simulink model "acquisition"  (R2020a)
settings: Solver=VariableStepAuto  StartTime=0.0  StopTime=simulation_time  RelTol=1e-3
values from neighbouring files (symbols this model uses):
  ca_fft_coef = zeros(37,4096)    [acquisition_hw_init.m]
  ca_fft_width = 14    [acquisition_hw_init.m]
  core_upsample_ratio = 24    [acquisition_hw_init.m]
  correlator_latency = 19    [acquisition_hw_init.m]
  ddc_latency = 5    [acquisition_hw_init.m]
  DDS_signal_width = 12    [acquisition_hw_init.m]
  f_start_phase = core_upsample_ratio*f_start/fs    (= -0.0006103515625)    [acquisition_hw_init.m]
  fd_phase_increment = core_upsample_ratio*(f_dds_change)/fs    (= 2e-05)    [acquisition_hw_init.m]
  fft_length = 4096    [acquisition_hw_init.m]
  fs = core_upsample_ratio*fs_adc    (= 120000000)    [acquisition_hw_init.m]
  ts = 1/fs    [acquisition_debugger_data.m]    (also in acquisition_hw_init.m = 8.33333333333e-09)
  ts_adc = 1/fs_adc    (= 2e-07)    [acquisition_hw_init.m]
libraries: xbsIndex_r4 x325
(part 2 of 2)

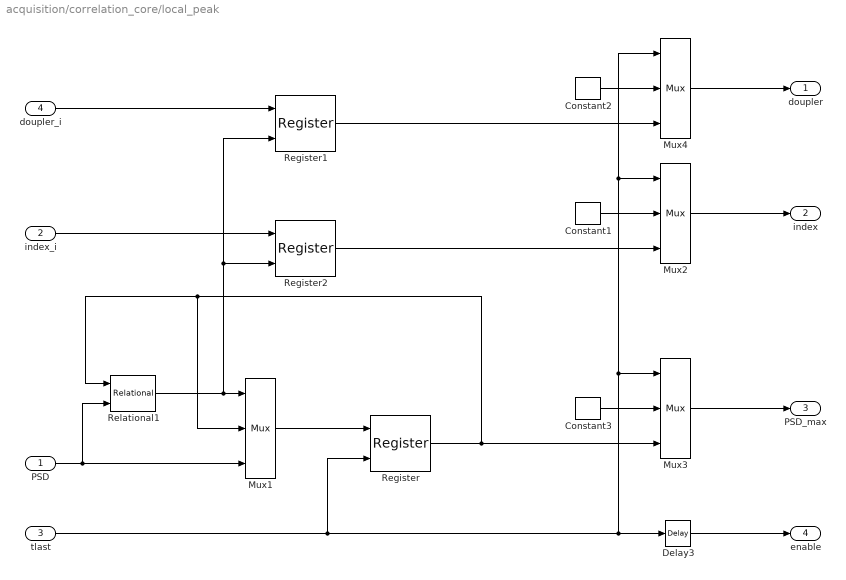
== system acquisition/correlation_core/local_peak ==
  PSD : Inport
  index_i : Inport  Port=2
  tlast : Inport  Port=3
  doupler_i : Inport  Port=4
  Constant1 : xbsIndex_r4/Constant  const=0  gui_display_data_type=Fixed-point  arith_type=Unsigned  n_bits=1  bin_pt=0  preci_type=Single  exp_width=8  frac_width=24  explicit_period=on  period=ts  equ=P=C  opselect=C  inp2=PCIN>>17  opr=+  inp1=P  carry=CIN  dbl_ovrd=off  block_type=constant
  Constant2 : xbsIndex_r4/Constant  const=0  gui_display_data_type=Fixed-point  arith_type=Unsigned  n_bits=DDS_phase_width  bin_pt=DDS_phase_width  preci_type=Single  exp_width=8  frac_width=24  explicit_period=on  period=ts  equ=P=C  opselect=C  inp2=PCIN>>17  opr=+  inp1=P  carry=CIN  dbl_ovrd=off  block_type=constant
  Constant3 : xbsIndex_r4/Constant  const=0  gui_display_data_type=Fixed-point  arith_type=Unsigned  n_bits=1  bin_pt=0  preci_type=Single  exp_width=8  frac_width=24  explicit_period=on  period=ts  equ=P=C  opselect=C  inp2=PCIN>>17  opr=+  inp1=P  carry=CIN  dbl_ovrd=off  block_type=constant
  Delay3 : xbsIndex_r4/Delay  rst=off  infoeditControl=Selection of Reset will increase slice count due to use of real FFs and instead of SRLs  en=off  latency=1  reg_retiming=off  dbl_ovrd=off  block_type=delay
  Mux1 : xbsIndex_r4/Mux  inputs=2  en=off  latency=0  precision=Full  arith_type=Unsigned  n_bits=16  bin_pt=14  quantization=Truncate  overflow=Wrap  dbl_ovrd=off  block_type=mux
  Mux2 : xbsIndex_r4/Mux  inputs=2  en=off  latency=1  precision=Full  arith_type=Unsigned  n_bits=16  bin_pt=14  quantization=Truncate  overflow=Wrap  dbl_ovrd=off  block_type=mux
  Mux3 : xbsIndex_r4/Mux  inputs=2  en=off  latency=1  precision=Full  arith_type=Unsigned  n_bits=16  bin_pt=14  quantization=Truncate  overflow=Wrap  dbl_ovrd=off  block_type=mux
  Mux4 : xbsIndex_r4/Mux  inputs=2  en=off  latency=1  precision=Full  arith_type=Unsigned  n_bits=16  bin_pt=14  quantization=Truncate  overflow=Wrap  dbl_ovrd=off  block_type=mux
  Register : xbsIndex_r4/Register  init=-2048  rst=on  en=off  dbl_ovrd=off  block_type=register
  Register1 : xbsIndex_r4/Register  init=0  rst=off  en=on  dbl_ovrd=off  block_type=register
  Register2 : xbsIndex_r4/Register  init=0  rst=off  en=on  dbl_ovrd=off  block_type=register
  Relational1 : xbsIndex_r4/Relational  mode=a<b  op_type=Bool  en=off  latency=0  dbl_ovrd=off  block_type=relational
  doupler : Outport
  index : Outport  Port=2
  PSD_max : Outport  Port=3
  enable : Outport  Port=4
  wires:
  Constant3/1 -> Mux3/2
  Constant1/1 -> Mux2/2
  Register2/1 -> Mux2/3
  Register/1 -> Relational1/1, Mux1/2, Mux3/3
  index_i/1 -> Register2/1
  Mux1/1 -> Register/1
  Relational1/1 -> Mux1/1, Register1/2, Register2/2
  PSD/1 -> Relational1/2, Mux1/3
  tlast/1 -> Register/2, Mux4/1, Mux2/1, Mux3/1, Delay3/1
  Delay3/1 -> enable/1
  Mux2/1 -> index/1
  Mux3/1 -> PSD_max/1
  doupler_i/1 -> Register1/1
  Constant2/1 -> Mux4/2
  Register1/1 -> Mux4/3
  Mux4/1 -> doupler/1

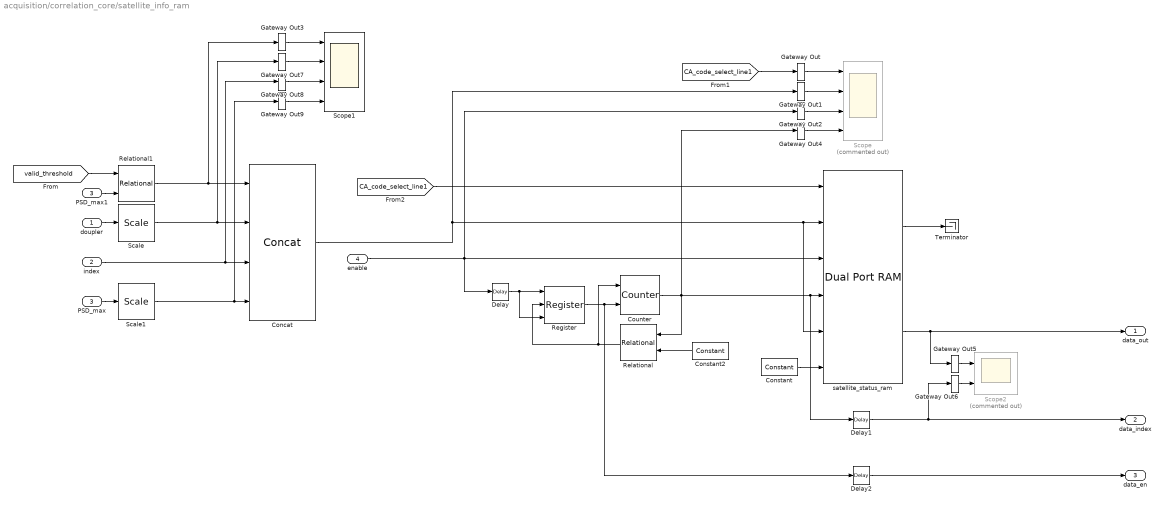
== system acquisition/correlation_core/satellite_info_ram ==
  doupler : Inport
  index : Inport  Port=2
  PSD_max : Inport  Port=3
  enable : Inport  Port=4
  Concat : xbsIndex_r4/Concat  num_inputs=4  dbl_ovrd=off  block_type=concat
  Constant : xbsIndex_r4/Constant  const=0  gui_display_data_type=Boolean  arith_type=Boolean  n_bits=16  bin_pt=14  preci_type=Single  exp_width=8  frac_width=24  explicit_period=on  period=ts  equ=P=C  opselect=C  inp2=PCIN>>17  opr=+  inp1=P  carry=CIN  dbl_ovrd=off  block_type=constant
  Constant2 : xbsIndex_r4/Constant  const=36  gui_display_data_type=Fixed-point  arith_type=Unsigned  n_bits=ceil(log2(37))  bin_pt=0  preci_type=Single  exp_width=8  frac_width=24  explicit_period=on  period=ts  equ=P=C  opselect=C  inp2=PCIN>>17  opr=+  inp1=P  carry=CIN  dbl_ovrd=off  block_type=constant
  Counter : xbsIndex_r4/Counter  cnt_type=Free Running  cnt_to=Inf  operation=Up  start_count=0  cnt_by_val=1  arith_type=Unsigned  n_bits=ceil(log2(37))  bin_pt=0  load_pin=off  rst=on  en=on  explicit_period=off  period=1  use_behavioral_HDL=off  implementation=Fabric  dbl_ovrd=off  block_type=counter
  Delay : xbsIndex_r4/Delay  rst=off  infoeditControl=Selection of Reset will increase slice count due to use of real FFs and instead of SRLs  en=off  latency=14  reg_retiming=off  dbl_ovrd=off  block_type=delay
  Delay1 : xbsIndex_r4/Delay  rst=off  infoeditControl=Selection of Reset will increase slice count due to use of real FFs and instead of SRLs  en=off  latency=1  reg_retiming=off  dbl_ovrd=off  block_type=delay
  Delay2 : xbsIndex_r4/Delay  rst=off  infoeditControl=Selection of Reset will increase slice count due to use of real FFs and instead of SRLs  en=off  latency=2  reg_retiming=off  dbl_ovrd=off  block_type=delay
  Gateway Out{,1..9} (10 alike) : xbsIndex_r4/Gateway Out  inherit_from_input=off  hdl_port=off  rows=1  columns=1  UseAsDAC=off  DACChannel='1'  interface=None  automatic_assignment=on  address_offset=hex2dec('00')  intf_name=''  intf_description=''  timing_constraint=None  locs_specified=off  LOCs={}  io_standard={}  block_type=gatewayout
  PSD_max1 : InportShadow  Port=3
  Register : xbsIndex_r4/Register  init=0  rst=on  en=on  dbl_ovrd=off  block_type=register
  Relational : xbsIndex_r4/Relational  mode=a>=b  op_type=Bool  en=off  latency=0  dbl_ovrd=off  block_type=relational
  Relational1 : xbsIndex_r4/Relational  mode=a<=b  op_type=Bool  en=off  latency=0  dbl_ovrd=off  block_type=relational
  Scale : xbsIndex_r4/Scale  scale_factor=DDS_phase_width  dbl_ovrd=off  block_type=scale
  Scale1 : xbsIndex_r4/Scale  scale_factor=abs_adder_point  dbl_ovrd=off  block_type=scale
  Scope : Scope  Commented=on  NumInputPorts=4
  Scope1 : Scope  NumInputPorts=4
  Scope2 : Scope  Commented=on  NumInputPorts=2
  Terminator : Terminator
  satellite_status_ram : xbsIndex_r4/Dual Port RAM  depth=37  initVector=1:37  distributed_mem=Block RAM  init_a=0  init_b=0  rst_a=off  rst_b=off  en_a=off  en_b=off  latency=1  write_mode_A=Read After Write  write_mode_B=Read After Write  optimize=Area  dbl_ovrd=off  simulation_type=fast_sim  block_type=dpram
  data_out : Outport
  data_index : Outport  Port=2
  data_en : Outport  Port=3
  wires:
  [CA_code_select_line1] -> satellite_status_ram/1
  PSD_max/1 -> Scale1/1
  enable/1 -> satellite_status_ram/3, Delay/1, Gateway Out2/1
  Scale/1 -> Gateway Out7/1, Concat/2
  doupler/1 -> Scale/1
  Gateway Out4/1 -> Scope/4
  Gateway Out1/1 -> Scope/2
  Gateway Out/1 -> Scope/1
  Gateway Out2/1 -> Scope/3
  [CA_code_select_line1] -> Gateway Out/1
  Constant/1 -> satellite_status_ram/6
  Concat/1 -> Gateway Out1/1, satellite_status_ram/5, satellite_status_ram/2
  Counter/1 -> Gateway Out4/1, Relational/1, Delay1/1, satellite_status_ram/4
  Register/1 -> Delay2/1, Counter/2
  Delay/1 -> Register/1, Register/3
  Relational/1 -> Counter/1, Register/2
  Constant2/1 -> Relational/2
  Gateway Out5/1 -> Scope2/1
  Gateway Out6/1 -> Scope2/2
  satellite_status_ram/2 -> data_out/1, Gateway Out5/1
  Delay1/1 -> data_index/1, Gateway Out6/1
  satellite_status_ram/1 -> Terminator/1
  Delay2/1 -> data_en/1
  index/1 -> Gateway Out8/1, Concat/3
  Scale1/1 -> Gateway Out9/1, Concat/4
  Relational1/1 -> Gateway Out3/1, Concat/1
  [valid_threshold] -> Relational1/1
  PSD_max1/1 -> Relational1/2
  Gateway Out8/1 -> Scope1/3
  Gateway Out3/1 -> Scope1/1
  Gateway Out7/1 -> Scope1/2
  Gateway Out9/1 -> Scope1/4

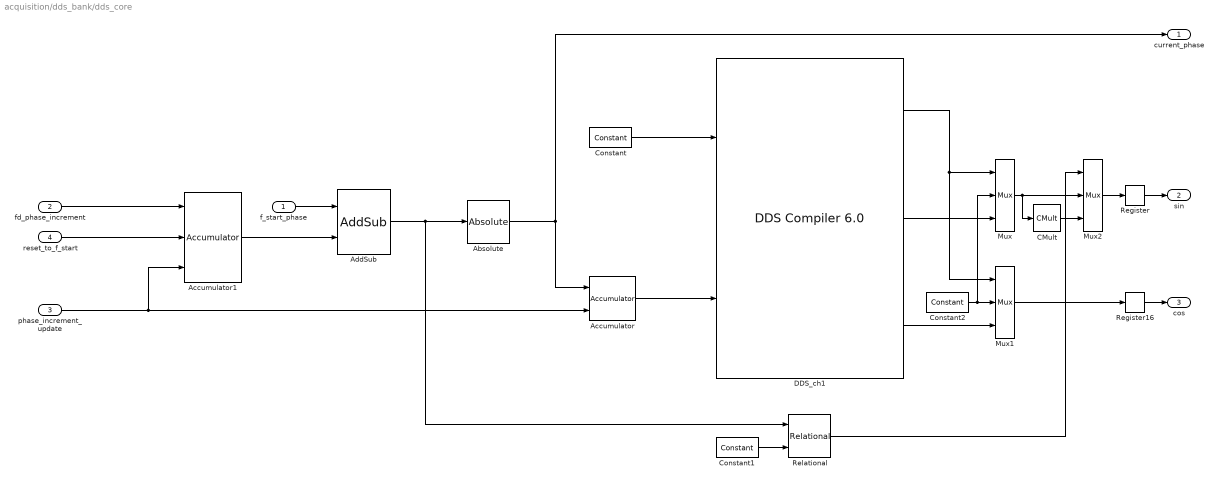
== system acquisition/dds_bank/dds_core ==
  f_start_phase : Inport
  fd_phase_increment : Inport  Port=2
  phase_increment_update : Inport  Port=3
  reset_to_f_start : Inport  Port=4
  Absolute : xbsIndex_r4/Absolute  precision=User Defined  arith_type=Unsigned  n_bits=DDS_phase_width  bin_pt=DDS_phase_width  quantization="Round  (unbiased: +/- Inf)"  overflow=Saturate  en=off  latency=0  dbl_ovrd=off  block_type=abs
  Accumulator : xbsIndex_r4/Accumulator  operation=Add  n_bits=DDS_phase_width  overflow=Wrap  scale=1  rst=on  hasbypass=off  infoeditControl=reset for floating point data type must be asserted for a minimum of 2 cycles  en=off  latency=1  msb_inp=100  msb=100  lsb=-100  use_behavioral_HDL=on  implementation=Fabric  dbl_ovrd=off  block_type=accum
  Accumulator1 : xbsIndex_r4/Accumulator  operation=Add  n_bits=DDS_phase_width  overflow=Wrap  scale=1  rst=on  hasbypass=off  infoeditControl=reset for floating point data type must be asserted for a minimum of 2 cycles  en=on  latency=1  msb_inp=100  msb=100  lsb=-100  use_behavioral_HDL=on  implementation=Fabric  dbl_ovrd=off  block_type=accum
  AddSub : xbsIndex_r4/AddSub  mode=Addition  use_carryin=off  use_carryout=off  en=off  latency=1  precision=Full  arith_type=Unsigned  n_bits=DDS_phase_width  bin_pt=DDS_phase_width  quantization="Round  (unbiased: +/- Inf)"  overflow=Saturate  use_behavioral_HDL=off  hw_selection=Fabric  pipelined=off  dbl_ovrd=off  block_type=addsub
  CMult : xbsIndex_r4/CMult  const=-1  gui_display_data_type=Fixed-point  const_n_bits=1  const_bin_pt=0  float_type=Single  exp_bits=8  fraction_bits=24  en=off  latency=0  precision=User Defined  arith_type="Signed  (2's comp)"  n_bits=DDS_signal_width  bin_pt=DDS_signal_width-1  quantization="Round  (unbiased: +/- Inf)"  overflow=Saturate  use_behavioral_HDL=off  mem_type=Distributed RAM  pipeline=off  dbl_ovrd=off  block_type=cmult
  Constant : xbsIndex_r4/Constant  const=1.0  gui_display_data_type=Boolean  arith_type=Boolean  n_bits=16  bin_pt=14  preci_type=Single  exp_width=8  frac_width=24  explicit_period=on  period=ts  equ=P=C  opselect=C  inp2=PCIN>>17  opr=+  inp1=P  carry=CIN  dbl_ovrd=off  block_type=constant
  Constant1 : xbsIndex_r4/Constant  const=0  gui_display_data_type=Fixed-point  arith_type=Unsigned  n_bits=1  bin_pt=0  preci_type=Single  exp_width=8  frac_width=24  explicit_period=on  period=ts  equ=P=C  opselect=C  inp2=PCIN>>17  opr=+  inp1=P  carry=CIN  dbl_ovrd=off  block_type=constant
  Constant2 : xbsIndex_r4/Constant  const=0  gui_display_data_type=Fixed-point  arith_type=Unsigned  n_bits=1  bin_pt=0  preci_type=Single  exp_width=8  frac_width=24  explicit_period=on  period=ts  equ=P=C  opselect=C  inp2=PCIN>>17  opr=+  inp1=P  carry=CIN  dbl_ovrd=off  block_type=constant
  DDS_ch1 : xbsIndex_r4/DDS Compiler 6.0   partspresent=SIN_COS_LUT_only  dds_clock_rate=100  channels=1  mode_of_operation=Standard  modulus=9  parameter_entry=Hardware_Parameters  spurious_free_dynamic_range=45  frequency_resolution=0.4  noise_shaping=Taylor_Series_Corrected  phase_width=DDS_phase_width  output_width=DDS_signal_width  output_selection=Sine_and_Cosine  negative_sine=off  negative_cosine=off  amplitude_mode=Full_Range  memory_type=Auto  optimization_goal=Auto  dsp48_use=Minimal  resync=off  latency_configuration=Auto  latency=1  has_phase_out=off  has_aclken=off  has_aresetn=off  explicit_period=off  period=1  data_has_tlast=Not_Required  has_tready=off  s_phase_has_tuser=Not_Required  m_data_has_tuser=Not_Required  m_phase_has_tuser=Not_Required  s_phase_tuser_width=1  output_form=Twos_Complement  s_config_sync_mode=On_Vector  phase_increment=Programmable  output_frequency1=0  output_frequency2=0  output_frequency3=0  output_frequency4=0  output_frequency5=0  output_frequency6=0  output_frequency7=0  output_frequency8=0  output_frequency9=0  output_frequency10=0  output_frequency11=0  output_frequency12=0  output_frequency13=0  output_frequency14=0  output_frequency15=0  output_frequency16=0  pinc1='0'  pinc2='0'  pinc3='0'  pinc4='0'  pinc5='0'  pinc6='0'  pinc7='0'  pinc8='0'  pinc9='0'  pinc10='0'  pinc11='0'  pinc12='0'  pinc13='0'  pinc14='0'  pinc15='0'  pinc16='0'  phase_offset=None  phase_offset_angles1=0  phase_offset_angles2=0  phase_offset_angles3=0  phase_offset_angles4=0  phase_offset_angles5=0  phase_offset_angles6=0  phase_offset_angles7=0  phase_offset_angles8=0  phase_offset_angles9=0  phase_offset_angles10=0  phase_offset_angles11=0  phase_offset_angles12=0  phase_offset_angles13=0  phase_offset_angles14=0  phase_offset_angles15=0  phase_offset_angles16=0  poff1='0'  poff2='0'  poff3='0'  poff4='0'  poff5='0'  poff6='0'  poff7='0'  poff8='0'  poff9='0'  poff10='0'  poff11='0'  poff12='0'  poff13='0'  poff14='0'  poff15='0'  poff16='0'  trim_axipin_name=on  simulation_type=hybrid_sim  simulation_model=sysgen:xddsv6_0_cmodel  data_path_portlist={ 's_axis_config_tdata_poff', 's_axis_config_tdata_chan0_poff', 's_axis_config_tdata_pinc', 's_axis_config_tdata_chan0_pinc', 's_axis_phase_tdata_resync', 's_axis_phase_tdata_chan0_resync', 's_axis_phase_tdata_poff', 's_axis_phase_tdata_chan0_poff', 's_axis_phase_tdata_pinc', 's_axis_phase_tdata_chan0_pinc', 's_axis_phase_tdata_phase_in', 'm_axis_data_tdata_sine', 'm_axis_data_tdata_chan0_sine', 'm_axis_data_tdata_cosine', 'm_axis_data_tdata_chan0_cosine', 'm_axis_phase_tdata_phase_out', 'm_axis_phase_tdata_chan0_phase_out'}  por_mode=false  gui_behaviour=Sysgen  ip_name=DDS Compiler  ip_version=6.0  dsptool_ready=true  wrapper_available=true  port_translation_map={ 'aclken' => 'en', 'aresetn' => 'rst' }  ipcore_usecache=true  ipcore_useipmodelcache=true  ipcore_xco_need_fpga_part=true  ipcore_verbose=false  block_type=dds_compiler_v6_0
  Mux : xbsIndex_r4/Mux  inputs=2  en=off  latency=1  precision=Full  arith_type=Unsigned  n_bits=16  bin_pt=14  quantization=Truncate  overflow=Wrap  dbl_ovrd=off  block_type=mux
  Mux1 : xbsIndex_r4/Mux  inputs=2  en=off  latency=1  precision=Full  arith_type=Unsigned  n_bits=16  bin_pt=14  quantization=Truncate  overflow=Wrap  dbl_ovrd=off  block_type=mux
  Mux2 : xbsIndex_r4/Mux  inputs=2  en=off  latency=0  precision=Full  arith_type=Unsigned  n_bits=16  bin_pt=14  quantization=Truncate  overflow=Wrap  dbl_ovrd=off  block_type=mux
  Register : xbsIndex_r4/Register  init=0  rst=off  en=off  dbl_ovrd=off  block_type=register
  Register16 : xbsIndex_r4/Register  init=0  rst=off  en=off  dbl_ovrd=off  block_type=register
  Relational : xbsIndex_r4/Relational  mode=a<b  op_type=Bool  en=off  latency=1  dbl_ovrd=off  block_type=relational
  current_phase : Outport
  sin : Outport  Port=2
  cos : Outport  Port=3
  wires:
  Mux/1 -> CMult/1, Mux2/2
  Mux1/1 -> Register16/1
  Constant/1 -> DDS_ch1/1
  reset_to_f_start/1 -> Accumulator1/2
  DDS_ch1/2 -> Mux/3
  DDS_ch1/3 -> Mux1/3
  Constant2/1 -> Mux/2, Mux1/2
  DDS_ch1/1 -> Mux1/1, Mux/1
  Accumulator/1 -> DDS_ch1/2
  phase_increment_update/1 -> Accumulator1/3, Accumulator/2
  AddSub/1 -> Relational/1, Absolute/1
  f_start_phase/1 -> AddSub/1
  fd_phase_increment/1 -> Accumulator1/1
  Accumulator1/1 -> AddSub/2
  Mux2/1 -> Register/1
  CMult/1 -> Mux2/3
  Constant1/1 -> Relational/2
  Absolute/1 -> Accumulator/1, current_phase/1
  Relational/1 -> Mux2/1
  Register/1 -> sin/1
  Register16/1 -> cos/1

== system acquisition/adc_dual_buffer/adc_addr_gen1/RE ==
  In : Inport
  Inverter : xbsIndex_r4/Inverter  en=off  latency=1  dbl_ovrd=off  block_type=inv
  Logical1 : xbsIndex_r4/Logical  logical_function=AND  inputs=2  en=off  latency=0  precision=Full  arith_type=Unsigned  n_bits=16  bin_pt=0  align_bp=on  dbl_ovrd=off  block_type=logical
  Out : Outport
  wires:
  Inverter/1 -> Logical1/2
  In/1 -> Inverter/1, Logical1/1
  Logical1/1 -> Out/1

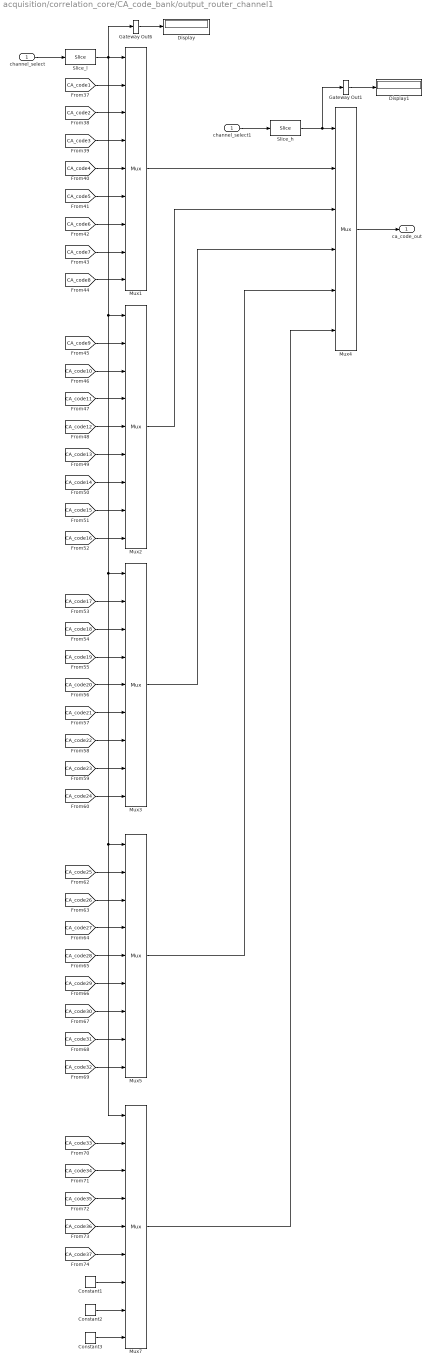
== system acquisition/correlation_core/CA_code_bank/output_router_channel1 ==
  channel_select : Inport
  Constant1 : xbsIndex_r4/Constant  const=0  gui_display_data_type=Fixed-point  arith_type=Unsigned  n_bits=1  bin_pt=0  preci_type=Single  exp_width=8  frac_width=24  explicit_period=on  period=ts  equ=P=C  opselect=C  inp2=PCIN>>17  opr=+  inp1=P  carry=CIN  dbl_ovrd=off  block_type=constant
  Constant2 : xbsIndex_r4/Constant  const=0  gui_display_data_type=Fixed-point  arith_type=Unsigned  n_bits=1  bin_pt=0  preci_type=Single  exp_width=8  frac_width=24  explicit_period=on  period=ts  equ=P=C  opselect=C  inp2=PCIN>>17  opr=+  inp1=P  carry=CIN  dbl_ovrd=off  block_type=constant
  Constant3 : xbsIndex_r4/Constant  const=0  gui_display_data_type=Fixed-point  arith_type=Unsigned  n_bits=1  bin_pt=0  preci_type=Single  exp_width=8  frac_width=24  explicit_period=on  period=ts  equ=P=C  opselect=C  inp2=PCIN>>17  opr=+  inp1=P  carry=CIN  dbl_ovrd=off  block_type=constant
  Display : Display
  Display1 : Display
  Gateway Out1 : xbsIndex_r4/Gateway Out  inherit_from_input=off  hdl_port=off  rows=1  columns=1  UseAsDAC=off  DACChannel='1'  interface=None  automatic_assignment=on  address_offset=hex2dec('00')  intf_name=''  intf_description=''  timing_constraint=None  locs_specified=off  LOCs={}  io_standard={}  block_type=gatewayout
  Gateway Out6 : xbsIndex_r4/Gateway Out  inherit_from_input=off  hdl_port=off  rows=1  columns=1  UseAsDAC=off  DACChannel='1'  interface=None  automatic_assignment=on  address_offset=hex2dec('00')  intf_name=''  intf_description=''  timing_constraint=None  locs_specified=off  LOCs={}  io_standard={}  block_type=gatewayout
  Mux{1..3,5,7} (5 alike) : xbsIndex_r4/Mux  inputs=8  en=off  latency=1  precision=Full  arith_type=Unsigned  n_bits=16  bin_pt=14  quantization=Truncate  overflow=Wrap  dbl_ovrd=off  block_type=mux
  Mux4 : xbsIndex_r4/Mux  inputs=5  en=off  latency=1  precision=Full  arith_type=Unsigned  n_bits=16  bin_pt=14  quantization=Truncate  overflow=Wrap  dbl_ovrd=off  block_type=mux
  Slice_h : xbsIndex_r4/Slice  nbits=3  boolean_output=off  mode=Lower Bit Location + Width  bit1=0  base1=MSB of Input  bit0=3  base0=LSB of Input  dbl_ovrd=off  block_type=slice
  Slice_l : xbsIndex_r4/Slice  nbits=3  boolean_output=off  mode=Lower Bit Location + Width  bit1=0  base1=MSB of Input  bit0=0  base0=LSB of Input  dbl_ovrd=off  block_type=slice
  channel_select1 : InportShadow
  ca_code_out : Outport
  wires:
  [CA_code10] -> Mux2/3
  [CA_code1] -> Mux1/2
  [CA_code18] -> Mux3/3
  [CA_code11] -> Mux2/4
  Mux7/1 -> Mux4/6
  [CA_code36] -> Mux7/5
  [CA_code16] -> Mux2/9
  [CA_code25] -> Mux5/2
  [CA_code3] -> Mux1/4
  [CA_code28] -> Mux5/5
  [CA_code33] -> Mux7/2
  [CA_code13] -> Mux2/6
  Mux2/1 -> Mux4/3
  [CA_code27] -> Mux5/4
  [CA_code35] -> Mux7/4
  [CA_code5] -> Mux1/6
  [CA_code4] -> Mux1/5
  [CA_code6] -> Mux1/7
  [CA_code8] -> Mux1/9
  [CA_code20] -> Mux3/5
  Mux4/1 -> ca_code_out/1
  [CA_code9] -> Mux2/2
  Mux3/1 -> Mux4/4
  [CA_code34] -> Mux7/3
  [CA_code22] -> Mux3/7
  [CA_code30] -> Mux5/7
  [CA_code37] -> Mux7/6
  [CA_code23] -> Mux3/8
  [CA_code19] -> Mux3/4
  [CA_code2] -> Mux1/3
  [CA_code24] -> Mux3/9
  [CA_code31] -> Mux5/8
  [CA_code26] -> Mux5/3
  Mux1/1 -> Mux4/2
  [CA_code21] -> Mux3/6
  Mux5/1 -> Mux4/5
  [CA_code29] -> Mux5/6
  [CA_code14] -> Mux2/7
  [CA_code12] -> Mux2/5
  [CA_code7] -> Mux1/8
  [CA_code15] -> Mux2/8
  [CA_code32] -> Mux5/9
  [CA_code17] -> Mux3/2
  Slice_l/1 -> Gateway Out6/1, Mux2/1, Mux3/1, Mux7/1, Mux5/1, Mux1/1
  channel_select/1 -> Slice_l/1
  channel_select1/1 -> Slice_h/1
  Slice_h/1 -> Gateway Out1/1, Mux4/1
  Gateway Out6/1 -> Display/1
  Gateway Out1/1 -> Display1/1
  Constant1/1 -> Mux7/7
  Constant2/1 -> Mux7/8
  Constant3/1 -> Mux7/9

== system acquisition/correlation_core/correlator_ch1/abs_pow2 ==
  a : Inport
  b : Inport  Port=2
  AddSub : xbsIndex_r4/AddSub  mode=Addition  use_carryin=off  use_carryout=off  en=off  latency=1  precision=User Defined  arith_type=Unsigned  n_bits=abs_adder_width  bin_pt=abs_adder_point  quantization="Round  (unbiased: +/- Inf)"  overflow=Saturate  use_behavioral_HDL=off  hw_selection=Fabric  pipelined=off  dbl_ovrd=off  block_type=addsub
  Mult8 : xbsIndex_r4/Mult  precision=User Defined  arith_type="Signed  (2's comp)"  n_bits=abs_multiplier_width  bin_pt=abs_multiplier_point  quantization="Round  (unbiased: +/- Inf)"  overflow=Saturate  en=off  latency=3  use_behavioral_HDL=off  opt=Speed  use_embedded=on  optimum_pipeline=off  pipeline=on  dbl_ovrd=off  use_rpm=on  placement_style=Triangular  block_type=mult
  Mult9 : xbsIndex_r4/Mult  precision=User Defined  arith_type="Signed  (2's comp)"  n_bits=abs_multiplier_width  bin_pt=abs_multiplier_point  quantization="Round  (unbiased: +/- Inf)"  overflow=Saturate  en=off  latency=3  use_behavioral_HDL=off  opt=Speed  use_embedded=on  optimum_pipeline=off  pipeline=on  dbl_ovrd=off  use_rpm=on  placement_style=Triangular  block_type=mult
  ap2_bp2 : Outport
  wires:
  b/1 -> Mult9/2, Mult9/1
  Mult8/1 -> AddSub/1
  a/1 -> Mult8/1, Mult8/2
  AddSub/1 -> ap2_bp2/1
  Mult9/1 -> AddSub/2

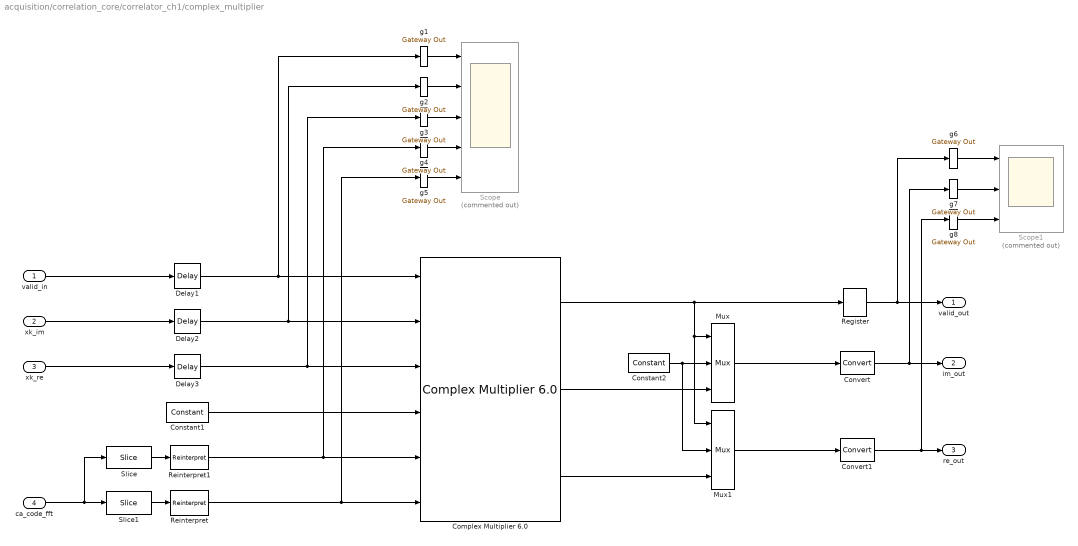
== system acquisition/correlation_core/correlator_ch1/complex_multiplier ==
  valid_in : Inport
  xk_im : Inport  Port=2
  xk_re : Inport  Port=3
  ca_code_fft : Inport  Port=4
  "Complex Multiplier 6.0 " : xbsIndex_r4/Complex Multiplier 6.0   hasatlast=off  hasatuser=off  atuserwidth=1  hasbtlast=off  hasbtuser=off  btuserwidth=1  multtype=Use_Mults  optimizegoal=Resources  flowcontrol=NonBlocking  outputwidth=cm_width  roundmode=Truncate  hasctrltlast=off  hasctrltuser=off  ctrltuserwidth=1  outtlastbehv=Null  latencyconfig=Automatic  minimumlatency=37  aclken=off  aresetn=off  trim_axipin_name=on  simulation_type=hybrid_sim  simulation_model=sysgen:cmpy_v6_0  data_path_portlist={ 's_axis_a_tdata_real', 's_axis_a_tdata_imag', 's_axis_b_tdata_real', 's_axis_b_tdata_imag', 's_axis_ctrl_tdata_rounding_bit', 'm_axis_dout_tdata_real', 'm_axis_dout_tdata_imag' }  aportwidth=63  bportwidth=63  ip_name=Complex Multiplier  ip_version=6.0  dsptool_ready=true  ipcore_usecache=true  ipcore_useipmodelcache=true  ipcore_verbose=false  ipcore_latency_parameter='minimumlatency'  wrapper_available=true  port_translation_map={ 'aclken' => 'en', 'aresetn' => 'rst'}  block_type=cmpy_v6_0
  Constant1 : xbsIndex_r4/Constant  const=1.0  gui_display_data_type=Boolean  arith_type=Boolean  n_bits=16  bin_pt=14  preci_type=Single  exp_width=8  frac_width=24  explicit_period=on  period=ts  equ=P=C  opselect=C  inp2=PCIN>>17  opr=+  inp1=P  carry=CIN  dbl_ovrd=off  block_type=constant
  Constant2 : xbsIndex_r4/Constant  const=0  gui_display_data_type=Fixed-point  arith_type=Unsigned  n_bits=1  bin_pt=0  preci_type=Single  exp_width=8  frac_width=24  explicit_period=on  period=ts  equ=P=C  opselect=C  inp2=PCIN>>17  opr=+  inp1=P  carry=CIN  dbl_ovrd=off  block_type=constant
  Convert : xbsIndex_r4/Convert  gui_display_data_type=Fixed-point  arith_type="Signed  (2's comp)"  n_bits=cm_convert_width  bin_pt=cm_convert_point  float_type=Single  exp_bits=8  fraction_bits=24  quantization="Round  (unbiased: +/- Inf)"  overflow=Saturate  en=off  latency=1  pipeline=off  dbl_ovrd=off  block_type=convert
  Convert1 : xbsIndex_r4/Convert  gui_display_data_type=Fixed-point  arith_type="Signed  (2's comp)"  n_bits=cm_convert_width  bin_pt=cm_convert_point  float_type=Single  exp_bits=8  fraction_bits=24  quantization="Round  (unbiased: +/- Inf)"  overflow=Saturate  en=off  latency=1  pipeline=off  dbl_ovrd=off  block_type=convert
  Delay1 : xbsIndex_r4/Delay  rst=off  infoeditControl=Selection of Reset will increase slice count due to use of real FFs and instead of SRLs  en=off  latency=ca_code_latency  reg_retiming=off  dbl_ovrd=off  block_type=delay
  Delay2 : xbsIndex_r4/Delay  rst=off  infoeditControl=Selection of Reset will increase slice count due to use of real FFs and instead of SRLs  en=off  latency=ca_code_latency  reg_retiming=off  dbl_ovrd=off  block_type=delay
  Delay3 : xbsIndex_r4/Delay  rst=off  infoeditControl=Selection of Reset will increase slice count due to use of real FFs and instead of SRLs  en=off  latency=ca_code_latency  reg_retiming=off  dbl_ovrd=off  block_type=delay
  Mux : xbsIndex_r4/Mux  inputs=2  en=off  latency=0  precision=Full  arith_type=Unsigned  n_bits=16  bin_pt=14  quantization=Truncate  overflow=Wrap  dbl_ovrd=off  block_type=mux
  Mux1 : xbsIndex_r4/Mux  inputs=2  en=off  latency=0  precision=Full  arith_type=Unsigned  n_bits=16  bin_pt=14  quantization=Truncate  overflow=Wrap  dbl_ovrd=off  block_type=mux
  Register : xbsIndex_r4/Register  init=0  rst=off  en=off  dbl_ovrd=off  block_type=register
  Reinterpret : xbsIndex_r4/Reinterpret  force_arith_type=on  arith_type="Signed  (2's comp)"  force_bin_pt=on  bin_pt=ca_fft_point  block_type=reinterpret
  Reinterpret1 : xbsIndex_r4/Reinterpret  force_arith_type=on  arith_type="Signed  (2's comp)"  force_bin_pt=on  bin_pt=ca_fft_point  block_type=reinterpret
  Scope : Scope  Commented=on  NumInputPorts=5
  Scope1 : Scope  Commented=on  NumInputPorts=3
  Slice : xbsIndex_r4/Slice  nbits=ca_fft_width  boolean_output=off  mode=Lower Bit Location + Width  bit1=0  base1=MSB of Input  bit0=0  base0=LSB of Input  dbl_ovrd=off  block_type=slice
  Slice1 : xbsIndex_r4/Slice  nbits=ca_fft_width  boolean_output=off  mode=Lower Bit Location + Width  bit1=0  base1=MSB of Input  bit0=ca_fft_width  base0=LSB of Input  dbl_ovrd=off  block_type=slice
  g{1..8} (8 alike) : xbsIndex_r4/Gateway Out  inherit_from_input=off  hdl_port=off  rows=1  columns=1  UseAsDAC=off  DACChannel='1'  interface=None  automatic_assignment=on  address_offset=hex2dec('00')  intf_name=''  intf_description=''  timing_constraint=None  locs_specified=off  LOCs={}  io_standard={}  block_type=gatewayout
  valid_out : Outport
  im_out : Outport  Port=2
  re_out : Outport  Port=3
  wires:
  Constant1/1 -> "Complex Multiplier 6.0 "/4
  Reinterpret/1 -> g5/1, "Complex Multiplier 6.0 "/6
  Reinterpret1/1 -> g4/1, "Complex Multiplier 6.0 "/5
  Slice/1 -> Reinterpret1/1
  Slice1/1 -> Reinterpret/1
  valid_in/1 -> Delay1/1
  xk_im/1 -> Delay2/1
  xk_re/1 -> Delay3/1
  "Complex Multiplier 6.0 "/1 -> Mux/1, Mux1/1, Register/1
  Mux/1 -> Convert/1
  Convert/1 -> g7/1, im_out/1
  Mux1/1 -> Convert1/1
  Convert1/1 -> g8/1, re_out/1
  "Complex Multiplier 6.0 "/2 -> Mux/3
  "Complex Multiplier 6.0 "/3 -> Mux1/3
  Constant2/1 -> Mux1/2, Mux/2
  g2/1 -> Scope/2
  g3/1 -> Scope/3
  g4/1 -> Scope/4
  g5/1 -> Scope/5
  g1/1 -> Scope/1
  g6/1 -> Scope1/1
  g7/1 -> Scope1/2
  g8/1 -> Scope1/3
  Register/1 -> g6/1, valid_out/1
  ca_code_fft/1 -> Slice1/1, Slice/1
  Delay1/1 -> g1/1, "Complex Multiplier 6.0 "/1
  Delay2/1 -> g2/1, "Complex Multiplier 6.0 "/2
  Delay3/1 -> g3/1, "Complex Multiplier 6.0 "/3

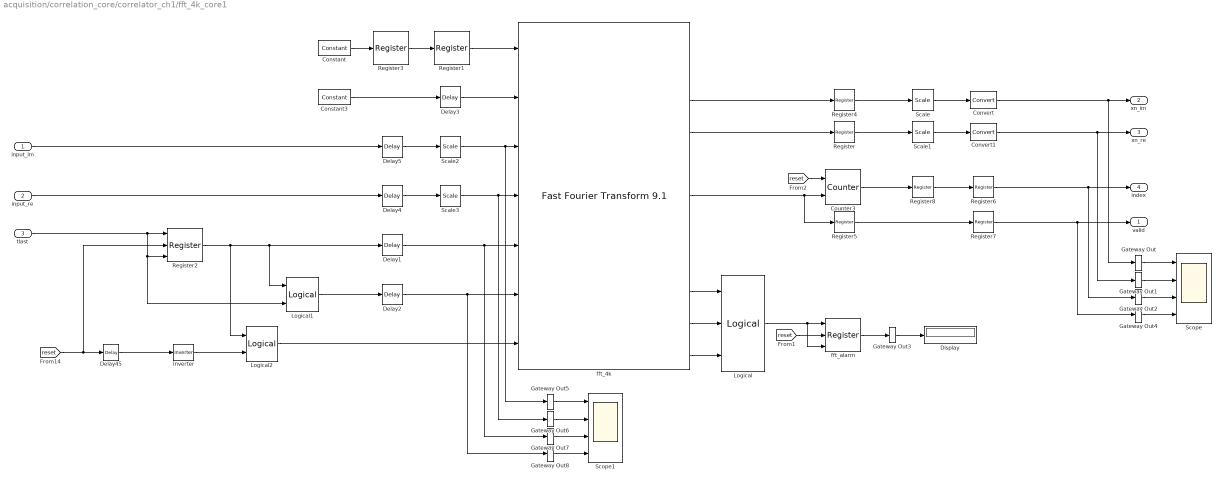
== system acquisition/correlation_core/correlator_ch1/fft_4k_core1 ==
  input_im : Inport
  input_re : Inport  Port=2
  tlast : Inport  Port=3
  Constant : xbsIndex_r4/Constant  const=1.0  gui_display_data_type=Fixed-point  arith_type=Unsigned  n_bits=1  bin_pt=0  preci_type=Single  exp_width=8  frac_width=24  explicit_period=on  period=ts  equ=P=C  opselect=C  inp2=PCIN>>17  opr=+  inp1=P  carry=CIN  dbl_ovrd=off  block_type=constant
  Constant3 : xbsIndex_r4/Constant  const=1.0  gui_display_data_type=Boolean  arith_type=Boolean  n_bits=16  bin_pt=14  preci_type=Single  exp_width=8  frac_width=24  explicit_period=on  period=ts  equ=P=C  opselect=C  inp2=PCIN>>17  opr=+  inp1=P  carry=CIN  dbl_ovrd=off  block_type=constant
  Convert : xbsIndex_r4/Convert  gui_display_data_type=Fixed-point  arith_type="Signed  (2's comp)"  n_bits=fft_convert_width  bin_pt=fft_convert_point  float_type=Single  exp_bits=8  fraction_bits=24  quantization="Round  (unbiased: +/- Inf)"  overflow=Saturate  en=off  latency=1  pipeline=off  dbl_ovrd=off  block_type=convert
  Convert1 : xbsIndex_r4/Convert  gui_display_data_type=Fixed-point  arith_type="Signed  (2's comp)"  n_bits=fft_convert_width  bin_pt=fft_convert_point  float_type=Single  exp_bits=8  fraction_bits=24  quantization="Round  (unbiased: +/- Inf)"  overflow=Saturate  en=off  latency=1  pipeline=off  dbl_ovrd=off  block_type=convert
  Counter3 : xbsIndex_r4/Counter  cnt_type=Free Running  cnt_to=Inf  operation=Up  start_count=0  cnt_by_val=1  arith_type=Unsigned  n_bits=ceil(log2(fft_length))  bin_pt=0  load_pin=off  rst=on  en=on  explicit_period=off  period=1  use_behavioral_HDL=off  implementation=Fabric  dbl_ovrd=off  block_type=counter
  Delay{1..5} (5 alike) : xbsIndex_r4/Delay  rst=off  infoeditControl=Selection of Reset will increase slice count due to use of real FFs and instead of SRLs  en=off  latency=3  reg_retiming=off  dbl_ovrd=off  block_type=delay
  Delay45 : xbsIndex_r4/Delay  rst=off  infoeditControl=Selection of Reset will increase slice count due to use of real FFs and instead of SRLs  en=off  latency=1  reg_retiming=off  dbl_ovrd=off  block_type=delay
  Display : Display
  Gateway Out{,1..8} (9 alike) : xbsIndex_r4/Gateway Out  inherit_from_input=off  hdl_port=off  rows=1  columns=1  UseAsDAC=off  DACChannel='1'  interface=None  automatic_assignment=on  address_offset=hex2dec('00')  intf_name=''  intf_description=''  timing_constraint=None  locs_specified=off  LOCs={}  io_standard={}  block_type=gatewayout
  Inverter : xbsIndex_r4/Inverter  en=off  latency=1  dbl_ovrd=off  block_type=inv
  Logical : xbsIndex_r4/Logical  logical_function=OR  inputs=3  en=off  latency=1  precision=Full  arith_type=Unsigned  n_bits=16  bin_pt=0  align_bp=on  dbl_ovrd=off  block_type=logical
  Logical1 : xbsIndex_r4/Logical  logical_function=AND  inputs=2  en=off  latency=1  precision=Full  arith_type=Unsigned  n_bits=16  bin_pt=0  align_bp=on  dbl_ovrd=off  block_type=logical
  Logical2 : xbsIndex_r4/Logical  logical_function=AND  inputs=2  en=off  latency=0  precision=Full  arith_type=Unsigned  n_bits=16  bin_pt=0  align_bp=on  dbl_ovrd=off  block_type=logical
  Register{,4..8} (6 alike) : xbsIndex_r4/Register  init=0  rst=off  en=off  dbl_ovrd=off  block_type=register
  Register1 : xbsIndex_r4/Register  init=1  rst=off  en=off  dbl_ovrd=off  block_type=register
  Register2 : xbsIndex_r4/Register  init=0  rst=on  en=on  dbl_ovrd=off  block_type=register
  Register3 : xbsIndex_r4/Register  init=1  rst=off  en=off  dbl_ovrd=off  block_type=register
  Scale : xbsIndex_r4/Scale  scale_factor=fft_output_scale  dbl_ovrd=off  block_type=scale
  Scale1 : xbsIndex_r4/Scale  scale_factor=fft_output_scale  dbl_ovrd=off  block_type=scale
  Scale2 : xbsIndex_r4/Scale  scale_factor=fft_input_scale  dbl_ovrd=off  block_type=scale
  Scale3 : xbsIndex_r4/Scale  scale_factor=fft_input_scale  dbl_ovrd=off  block_type=scale
  Scope : Scope  NumInputPorts=4
  Scope1 : Scope  NumInputPorts=4
  fft_4k : xbsIndex_r4/Fast Fourier Transform 9.1   transform_length=4096  target_clock_frequency=fs*1e-6  target_data_throughput=50  implementation_options=pipelined_streaming_io  run_time_configurable_transform_length=off  phase_factor_width=24  scaling_options=unscaled  rounding_modes=convergent_rounding  aclken=off  aresetn=on  output_ordering=natural_order  cyclic_prefix_insertion=off  throttle_scheme=realtime  xk_index=on  ovflo=off  trim_axipin_name=on  memory_options_data=block_ram  memory_options_phase_factors=block_ram  number_of_stages_using_block_ram_for_data_and_phase_factors=5  memory_options_reorder=block_ram  memory_options_hybrid=on  complex_mult_type=use_mults_resources  butterfly_type=use_xtremedsp_slices  simulation_type=hybrid_sim  simulation_model=sysgen:xfftv9_cmodel  data_path_portlist={ 's_axis_data_tdata', 'm_axis_data_tdata', 'm_axis_status_tdata', 'event_fft_overflow' }  channels=1  input_ordering=natural_order  input_width=16  ip_name=Fast Fourier Transform  ip_version=9.1  dsptool_ready=true  ipcore_usecache=true  ipcore_useipmodelcache=true  wrapper_available=true  port_translation_map={ 'aclken' => 'en', 'aresetn' => 'rst'}  data_format=fixed_point  block_type=xfft_v9_1
  fft_alarm : xbsIndex_r4/Register  init=0  rst=on  en=on  dbl_ovrd=off  block_type=register
  valid : Outport
  xn_im : Outport  Port=2
  xn_re : Outport  Port=3
  index : Outport  Port=4
  wires:
  Logical1/1 -> Delay2/1
  Delay3/1 -> fft_4k/2
  tlast/1 -> Logical1/2, Register2/3, Register2/1
  Logical2/1 -> fft_4k/7
  Register2/1 -> Logical1/1, Delay1/1, Logical2/1
  fft_4k/3 -> Register4/1
  [reset] -> Register2/2, Delay45/1
  Constant/1 -> Register3/1
  Delay45/1 -> Inverter/1
  Inverter/1 -> Logical2/2
  fft_4k/4 -> Register/1
  Delay1/1 -> Gateway Out7/1, fft_4k/5
  Delay2/1 -> Gateway Out8/1, fft_4k/6
  Register1/1 -> fft_4k/1
  Register3/1 -> Register1/1
  Constant3/1 -> Delay3/1
  fft_4k/9 -> Logical/1
  fft_4k/10 -> Logical/2
  fft_4k/11 -> Logical/3
  Logical/1 -> fft_alarm/3, fft_alarm/1
  [reset] -> fft_alarm/2
  [reset] -> Counter3/1
  fft_4k/6 -> Register5/1, Counter3/2
  Counter3/1 -> Register8/1
  Register/1 -> Scale1/1
  Register4/1 -> Scale/1
  fft_alarm/1 -> Gateway Out3/1
  Register5/1 -> Register7/1
  Scale/1 -> Convert/1
  Scale1/1 -> Convert1/1
  Convert/1 -> xn_im/1, Gateway Out/1
  Register6/1 -> Gateway Out2/1, index/1
  Register7/1 -> Gateway Out4/1, valid/1
  Convert1/1 -> Gateway Out1/1, xn_re/1
  Gateway Out/1 -> Scope/1
  Gateway Out1/1 -> Scope/2
  Gateway Out3/1 -> Display/1
  Gateway Out4/1 -> Scope/4
  Gateway Out2/1 -> Scope/3
  input_im/1 -> Delay5/1
  input_re/1 -> Delay4/1
  Scale2/1 -> Gateway Out5/1, fft_4k/3
  Scale3/1 -> Gateway Out6/1, fft_4k/4
  Delay4/1 -> Scale3/1
  Delay5/1 -> Scale2/1
  Register8/1 -> Register6/1
  Gateway Out7/1 -> Scope1/3
  Gateway Out8/1 -> Scope1/4
  Gateway Out6/1 -> Scope1/2
  Gateway Out5/1 -> Scope1/1

== system acquisition/correlation_core/correlator_ch1/fine_acquisition_integrator ==
  ap2_bp2 : Inport
  index : Inport  Port=2
  tlast : Inport  Port=3
  abs_out : Outport
  index_out : Outport  Port=2
  tlast_out : Outport  Port=3
  wires:
  index/1 -> index_out/1
  ap2_bp2/1 -> abs_out/1
  tlast/1 -> tlast_out/1

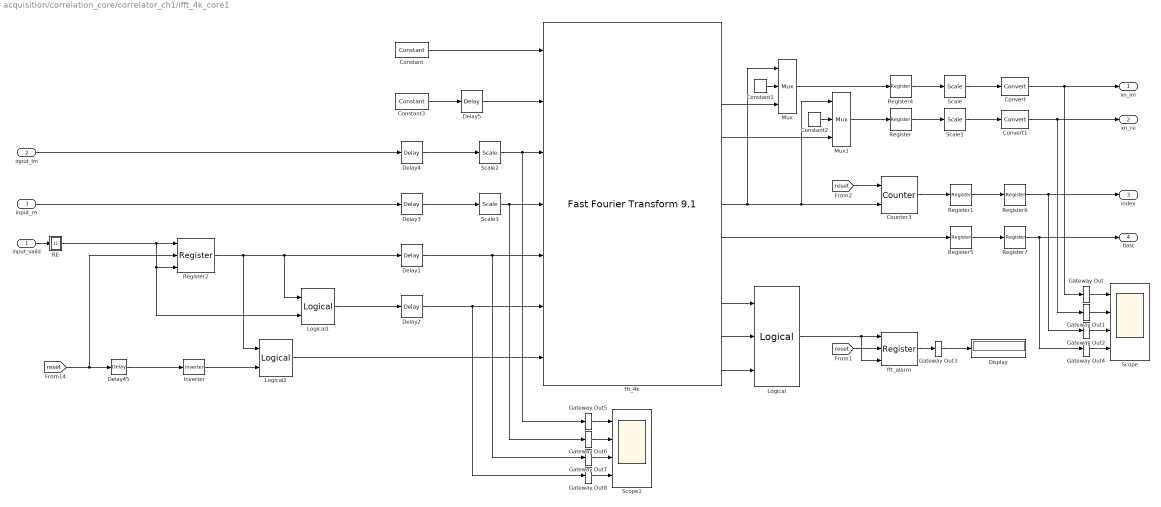
== system acquisition/correlation_core/correlator_ch1/ifft_4k_core1 ==
  input_valid : Inport
  input_im : Inport  Port=2
  input_re : Inport  Port=3
  Constant : xbsIndex_r4/Constant  const=0  gui_display_data_type=Fixed-point  arith_type=Unsigned  n_bits=1  bin_pt=0  preci_type=Single  exp_width=8  frac_width=24  explicit_period=on  period=ts  equ=P=C  opselect=C  inp2=PCIN>>17  opr=+  inp1=P  carry=CIN  dbl_ovrd=off  block_type=constant
  Constant1 : xbsIndex_r4/Constant  const=0  gui_display_data_type=Fixed-point  arith_type=Unsigned  n_bits=1  bin_pt=0  preci_type=Single  exp_width=8  frac_width=24  explicit_period=on  period=ts  equ=P=C  opselect=C  inp2=PCIN>>17  opr=+  inp1=P  carry=CIN  dbl_ovrd=off  block_type=constant
  Constant2 : xbsIndex_r4/Constant  const=0  gui_display_data_type=Fixed-point  arith_type=Unsigned  n_bits=1  bin_pt=0  preci_type=Single  exp_width=8  frac_width=24  explicit_period=on  period=ts  equ=P=C  opselect=C  inp2=PCIN>>17  opr=+  inp1=P  carry=CIN  dbl_ovrd=off  block_type=constant
  Constant3 : xbsIndex_r4/Constant  const=1.0  gui_display_data_type=Boolean  arith_type=Boolean  n_bits=16  bin_pt=14  preci_type=Single  exp_width=8  frac_width=24  explicit_period=on  period=ts  equ=P=C  opselect=C  inp2=PCIN>>17  opr=+  inp1=P  carry=CIN  dbl_ovrd=off  block_type=constant
  Convert : xbsIndex_r4/Convert  gui_display_data_type=Fixed-point  arith_type="Signed  (2's comp)"  n_bits=ifft_convert_width  bin_pt=ifft_convert_point  float_type=Single  exp_bits=8  fraction_bits=24  quantization="Round  (unbiased: +/- Inf)"  overflow=Saturate  en=off  latency=1  pipeline=off  dbl_ovrd=off  block_type=convert
  Convert1 : xbsIndex_r4/Convert  gui_display_data_type=Fixed-point  arith_type="Signed  (2's comp)"  n_bits=ifft_convert_width  bin_pt=ifft_convert_point  float_type=Single  exp_bits=8  fraction_bits=24  quantization="Round  (unbiased: +/- Inf)"  overflow=Saturate  en=off  latency=1  pipeline=off  dbl_ovrd=off  block_type=convert
  Counter3 : xbsIndex_r4/Counter  cnt_type=Free Running  cnt_to=Inf  operation=Up  start_count=0  cnt_by_val=1  arith_type=Unsigned  n_bits=ceil(log2(fft_length))  bin_pt=0  load_pin=off  rst=on  en=on  explicit_period=off  period=1  use_behavioral_HDL=off  implementation=Fabric  dbl_ovrd=off  block_type=counter
  Delay{1..5} (5 alike) : xbsIndex_r4/Delay  rst=off  infoeditControl=Selection of Reset will increase slice count due to use of real FFs and instead of SRLs  en=off  latency=3  reg_retiming=off  dbl_ovrd=off  block_type=delay
  Delay45 : xbsIndex_r4/Delay  rst=off  infoeditControl=Selection of Reset will increase slice count due to use of real FFs and instead of SRLs  en=off  latency=1  reg_retiming=off  dbl_ovrd=off  block_type=delay
  Display : Display
  Gateway Out{,1..8} (9 alike) : xbsIndex_r4/Gateway Out  inherit_from_input=off  hdl_port=off  rows=1  columns=1  UseAsDAC=off  DACChannel='1'  interface=None  automatic_assignment=on  address_offset=hex2dec('00')  intf_name=''  intf_description=''  timing_constraint=None  locs_specified=off  LOCs={}  io_standard={}  block_type=gatewayout
  Inverter : xbsIndex_r4/Inverter  en=off  latency=1  dbl_ovrd=off  block_type=inv
  Logical : xbsIndex_r4/Logical  logical_function=OR  inputs=3  en=off  latency=1  precision=Full  arith_type=Unsigned  n_bits=16  bin_pt=0  align_bp=on  dbl_ovrd=off  block_type=logical
  Logical1 : xbsIndex_r4/Logical  logical_function=AND  inputs=2  en=off  latency=1  precision=Full  arith_type=Unsigned  n_bits=16  bin_pt=0  align_bp=on  dbl_ovrd=off  block_type=logical
  Logical2 : xbsIndex_r4/Logical  logical_function=AND  inputs=2  en=off  latency=0  precision=Full  arith_type=Unsigned  n_bits=16  bin_pt=0  align_bp=on  dbl_ovrd=off  block_type=logical
  Mux : xbsIndex_r4/Mux  inputs=2  en=off  latency=0  precision=Full  arith_type=Unsigned  n_bits=16  bin_pt=14  quantization=Truncate  overflow=Wrap  dbl_ovrd=off  block_type=mux
  Mux1 : xbsIndex_r4/Mux  inputs=2  en=off  latency=0  precision=Full  arith_type=Unsigned  n_bits=16  bin_pt=14  quantization=Truncate  overflow=Wrap  dbl_ovrd=off  block_type=mux
  RE : Subsystem
  Register{,1,4..7} (6 alike) : xbsIndex_r4/Register  init=0  rst=off  en=off  dbl_ovrd=off  block_type=register
  Register2 : xbsIndex_r4/Register  init=0  rst=on  en=on  dbl_ovrd=off  block_type=register
  Scale : xbsIndex_r4/Scale  scale_factor=ifft_output_scale  dbl_ovrd=off  block_type=scale
  Scale1 : xbsIndex_r4/Scale  scale_factor=ifft_output_scale  dbl_ovrd=off  block_type=scale
  Scale2 : xbsIndex_r4/Scale  scale_factor=ifft_input_scale  dbl_ovrd=off  block_type=scale
  Scale3 : xbsIndex_r4/Scale  scale_factor=ifft_input_scale  dbl_ovrd=off  block_type=scale
  Scope : Scope  NumInputPorts=4
  Scope1 : Scope  NumInputPorts=4
  fft_4k : xbsIndex_r4/Fast Fourier Transform 9.1   transform_length=4096  target_clock_frequency=fs*1e-6  target_data_throughput=50  implementation_options=pipelined_streaming_io  run_time_configurable_transform_length=off  phase_factor_width=16  scaling_options=unscaled  rounding_modes=convergent_rounding  aclken=off  aresetn=on  output_ordering=natural_order  cyclic_prefix_insertion=off  throttle_scheme=realtime  xk_index=on  ovflo=off  trim_axipin_name=off  memory_options_data=block_ram  memory_options_phase_factors=block_ram  number_of_stages_using_block_ram_for_data_and_phase_factors=5  memory_options_reorder=block_ram  memory_options_hybrid=on  complex_mult_type=use_mults_resources  butterfly_type=use_luts  simulation_type=hybrid_sim  simulation_model=sysgen:xfftv9_cmodel  data_path_portlist={ 's_axis_data_tdata', 'm_axis_data_tdata', 'm_axis_status_tdata', 'event_fft_overflow' }  channels=1  input_ordering=natural_order  input_width=16  ip_name=Fast Fourier Transform  ip_version=9.1  dsptool_ready=true  ipcore_usecache=true  ipcore_useipmodelcache=true  wrapper_available=true  port_translation_map={ 'aclken' => 'en', 'aresetn' => 'rst'}  data_format=fixed_point  block_type=xfft_v9_1
  fft_alarm : xbsIndex_r4/Register  init=0  rst=on  en=on  dbl_ovrd=off  block_type=register
  xn_im : Outport
  xn_re : Outport  Port=2
  index : Outport  Port=3
  tlast : Outport  Port=4
  wires:
  Register5/1 -> Register7/1
  fft_alarm/1 -> Gateway Out3/1
  Register4/1 -> Scale/1
  Register/1 -> Scale1/1
  Counter3/1 -> Register1/1
  fft_4k/6 -> Mux/1, Counter3/2, Mux1/1
  [reset] -> Counter3/1
  [reset] -> fft_alarm/2
  Logical/1 -> fft_alarm/1, fft_alarm/3
  fft_4k/11 -> Logical/3
  fft_4k/10 -> Logical/2
  fft_4k/9 -> Logical/1
  Constant/1 -> fft_4k/1
  Delay2/1 -> Gateway Out8/1, fft_4k/6
  Delay1/1 -> Gateway Out7/1, fft_4k/5
  Inverter/1 -> Logical2/2
  Delay45/1 -> Inverter/1
  input_im/1 -> Delay4/1
  [reset] -> Delay45/1, Register2/2
  fft_4k/3 -> Mux/3
  Logical2/1 -> fft_4k/7
  input_valid/1 -> RE/1(In)
  Register2/1 -> Logical2/1, Delay1/1, Logical1/1
  Logical1/1 -> Delay2/1
  RE/1(Out) -> Register2/1, Register2/3, Logical1/2
  fft_4k/7 -> Register5/1
  Scale/1 -> Convert/1
  Convert/1 -> xn_im/1, Gateway Out/1
  Convert1/1 -> xn_re/1, Gateway Out1/1
  Scale1/1 -> Convert1/1
  Register6/1 -> index/1, Gateway Out2/1
  Register7/1 -> Gateway Out4/1, tlast/1
  input_re/1 -> Delay3/1
  Gateway Out/1 -> Scope/1
  Gateway Out1/1 -> Scope/2
  Gateway Out2/1 -> Scope/3
  Gateway Out4/1 -> Scope/4
  Gateway Out3/1 -> Display/1
  Mux/1 -> Register4/1
  fft_4k/4 -> Mux1/3
  Mux1/1 -> Register/1
  Constant1/1 -> Mux/2
  Constant2/1 -> Mux1/2
  Delay3/1 -> Scale3/1
  Delay4/1 -> Scale2/1
  Scale2/1 -> Gateway Out5/1, fft_4k/3
  Scale3/1 -> Gateway Out6/1, fft_4k/4
  Register1/1 -> Register6/1
  Gateway Out8/1 -> Scope1/4
  Gateway Out7/1 -> Scope1/3
  Gateway Out6/1 -> Scope1/2
  Gateway Out5/1 -> Scope1/1
  Delay5/1 -> fft_4k/2
  Constant3/1 -> Delay5/1

== system acquisition/correlation_core/correlator_ch1/local_peak ==
  PSD : Inport
  index_i : Inport  Port=2
  tlast : Inport  Port=3
  Constant1 : xbsIndex_r4/Constant  const=0  gui_display_data_type=Fixed-point  arith_type=Unsigned  n_bits=1  bin_pt=0  preci_type=Single  exp_width=8  frac_width=24  explicit_period=on  period=ts  equ=P=C  opselect=C  inp2=PCIN>>17  opr=+  inp1=P  carry=CIN  dbl_ovrd=off  block_type=constant
  Constant3 : xbsIndex_r4/Constant  const=0  gui_display_data_type=Fixed-point  arith_type=Unsigned  n_bits=1  bin_pt=0  preci_type=Single  exp_width=8  frac_width=24  explicit_period=on  period=ts  equ=P=C  opselect=C  inp2=PCIN>>17  opr=+  inp1=P  carry=CIN  dbl_ovrd=off  block_type=constant
  Delay3 : xbsIndex_r4/Delay  rst=off  infoeditControl=Selection of Reset will increase slice count due to use of real FFs and instead of SRLs  en=off  latency=1  reg_retiming=off  dbl_ovrd=off  block_type=delay
  Mux1 : xbsIndex_r4/Mux  inputs=2  en=off  latency=0  precision=Full  arith_type=Unsigned  n_bits=16  bin_pt=14  quantization=Truncate  overflow=Wrap  dbl_ovrd=off  block_type=mux
  Mux2 : xbsIndex_r4/Mux  inputs=2  en=off  latency=1  precision=Full  arith_type=Unsigned  n_bits=16  bin_pt=14  quantization=Truncate  overflow=Wrap  dbl_ovrd=off  block_type=mux
  Mux3 : xbsIndex_r4/Mux  inputs=2  en=off  latency=1  precision=Full  arith_type=Unsigned  n_bits=16  bin_pt=14  quantization=Truncate  overflow=Wrap  dbl_ovrd=off  block_type=mux
  Register : xbsIndex_r4/Register  init=-2048  rst=on  en=off  dbl_ovrd=off  block_type=register
  Register2 : xbsIndex_r4/Register  init=0  rst=off  en=on  dbl_ovrd=off  block_type=register
  Relational1 : xbsIndex_r4/Relational  mode=a<b  op_type=Bool  en=off  latency=0  dbl_ovrd=off  block_type=relational
  PSD_max : Outport
  index : Outport  Port=2
  enable : Outport  Port=3
  wires:
  Constant3/1 -> Mux3/2
  Constant1/1 -> Mux2/2
  Register2/1 -> Mux2/3
  Register/1 -> Relational1/1, Mux1/2, Mux3/3
  index_i/1 -> Register2/1
  Mux1/1 -> Register/1
  Relational1/1 -> Mux1/1, Register2/2
  PSD/1 -> Relational1/2, Mux1/3
  tlast/1 -> Register/2, Delay3/1, Mux2/1, Mux3/1
  Delay3/1 -> enable/1
  Mux2/1 -> index/1
  Mux3/1 -> PSD_max/1

== system acquisition/correlation_core/correlator_ch1/ifft_4k_core1/RE ==
  In : Inport
  Inverter : xbsIndex_r4/Inverter  en=off  latency=1  dbl_ovrd=off  block_type=inv
  Logical1 : xbsIndex_r4/Logical  logical_function=AND  inputs=2  en=off  latency=0  precision=Full  arith_type=Unsigned  n_bits=16  bin_pt=0  align_bp=on  dbl_ovrd=off  block_type=logical
  Out : Outport
  wires:
  Inverter/1 -> Logical1/2
  In/1 -> Inverter/1, Logical1/1
  Logical1/1 -> Out/1
